simulink model "bicycle_kin_sim"  (R2020b)
settings: Solver=FixedStepAuto  StartTime=0.0  StopTime=inf  FixedStep=0.01  RelTol=1e-3
libraries: robotlib x8
settings Model: Creator=bascetta  LastModifiedBy=root
settings OptimizationCC: EnhancedBackFolding=on  PassReuseOutputArgsAs=Individual arguments  ZeroExternalMemoryAtStartup=off  ZeroInternalMemoryAtStartup=off  MaxStackSize=64  OptimizeBlockOrder=speed  DifferentSizesBufferReuse=on  OptimizationCustomize=off  EfficientTunableParamExpr=on
settings DebuggingCC: ParameterTunabilityLossMsg=error
settings HardwareCC: ProdBitPerPointer=32  ProdBitPerSizeT=32  ProdBitPerPtrDiffT=32  ProdLargestAtomicFloat=None  ProdIntDivRoundTo=Undefined  ProdEndianess=Unspecified  ProdWordSize=32  ProdHWDeviceType=Generic->Unspecified (assume 32-bit Generic)
settings SFSimCC: MATLABDynamicMemAlloc=off  SimTargetLang=C++
settings RTWCC: Description=Embedded Coder  SystemTargetFile=ert.tlc  HardwareBoard=Robot Operating System (ROS)  TLCOptions="-aInlineSetEventsForThisBaseRateFcn=TLC_FALSE -aSuppressMultiTaskScheduler=TLC_FALSE  -aRateBasedStepFcn=0"  GenCodeOnly=on  TemplateMakefile=ert_default_tmf  Toolchain=Catkin  TargetLang=C++
settings CodeAppCC: ForceParamTrailComments=on  IgnoreCustomStorageClasses=off  OperatorAnnotations=on  SimulinkDataObjDesc=on  SFDataObjDesc=on  InsertBlockDesc=on
settings ERTTargetCC: SupportContinuousTime=on  SupportVariableSizeSignals=on

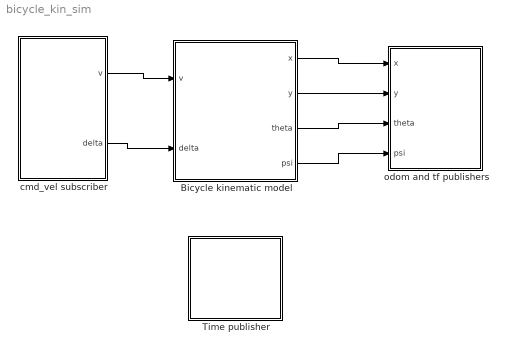
== system bicycle_kin_sim ==
  Bicycle kinematic model : Subsystem  mask{state0=[88, 182, 3.93], RCD=1.6, CFD=1.1}
      mask prompts: state0 "Initial conditions (x0, y0, theta0)"; RCD "Rear-Centre Distance"; CFD "Centre-Front Distance"
      mask TypeOptions RCD: Rear-Centre Distance/Value
      mask TypeOptions CFD: Centre-Front Distance/Value
  Time publisher : Subsystem
  cmd_vel subscriber : Subsystem
  odom and tf publishers : Subsystem  mask{simPublishRate=100}
      mask prompts: simPublishRate "Publising rate [Hz]"
  wires:
  Bicycle kinematic model/1(x) -> odom and tf publishers/1(x)
  Bicycle kinematic model/2(y) -> odom and tf publishers/2(y)
  Bicycle kinematic model/3(theta) -> odom and tf publishers/3(theta)
  cmd_vel subscriber/1(v) -> Bicycle kinematic model/1(v)
  cmd_vel subscriber/2(delta) -> Bicycle kinematic model/2(delta)
  Bicycle kinematic model/4(psi) -> odom and tf publishers/4(psi)

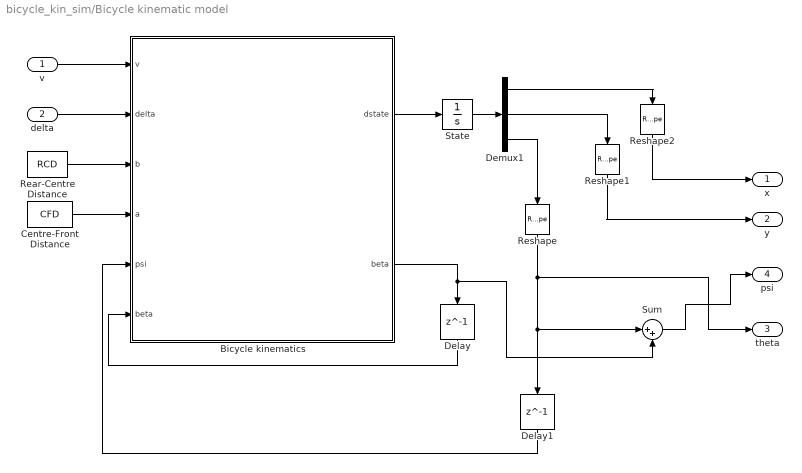
== system bicycle_kin_sim/Bicycle kinematic model ==
  v : Inport
  delta : Inport  Port=2
  Bicycle kinematics : MATLAB Function  TreatAsAtomicUnit=on
  Centre-Front Distance : Constant  Value=CFD
  Delay : Delay  DelayLength=1  InitialCondition=0
  Delay1 : Delay  DelayLength=1  InitialCondition=0
  Demux1 : Demux  Outputs=3
  Rear-Centre Distance : Constant  Value=RCD
  Reshape : Reshape
  Reshape1 : Reshape
  Reshape2 : Reshape
  State : Integrator  InitialCondition=state0
  Sum : Sum  Inputs=|++
  x : Outport  VectorParamsAs1DForOutWhenUnconnected=off
  y : Outport  Port=2  VectorParamsAs1DForOutWhenUnconnected=off
  theta : Outport  Port=3  VectorParamsAs1DForOutWhenUnconnected=off
  psi : Outport  Port=4  VectorParamsAs1DForOutWhenUnconnected=off
  wires:
  Bicycle kinematics/1(dstate) -> State/1
  State/1 -> Demux1/1
  Demux1/2 -> Reshape1/1
  Demux1/1 -> Reshape2/1
  delta/1 -> Bicycle kinematics/2(delta)
  v/1 -> Bicycle kinematics/1(v)
  Demux1/3 -> Reshape/1
  Bicycle kinematics/2(beta) -> Sum/2, Delay/1
  Rear-Centre Distance/1 -> Bicycle kinematics/3(b)
  Centre-Front Distance/1 -> Bicycle kinematics/4(a)
  Delay/1 -> Bicycle kinematics/6("beta ")
  Delay1/1 -> Bicycle kinematics/5(psi)
  Reshape/1 -> theta/1, Sum/1, Delay1/1
  Reshape1/1 -> y/1
  Reshape2/1 -> x/1
  Sum/1 -> psi/1

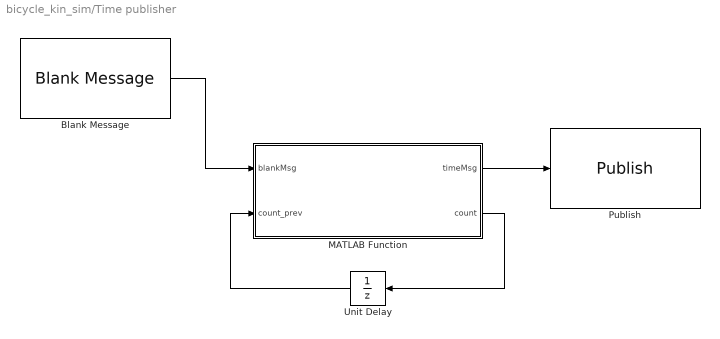
== system bicycle_kin_sim/Time publisher ==
  Blank Message : robotlib/Blank Message  messageClass=Message  entityType=rosgraph_msgs/Clock  messageType=rosgraph_msgs/Clock  SampleTime=0.01  legacyBusStruct=off
  MATLAB Function : MATLAB Function  TreatAsAtomicUnit=on
  Publish : robotlib/Publish  topicSource=Specify your own  topic=/clock  messageType=rosgraph_msgs/Clock  legacyBusStruct=off  messageQueueLength=1
  Unit Delay : UnitDelay  SampleTime=0.01  HasFrameUpgradeWarning=on
  wires:
  MATLAB Function/1(timeMsg) -> Publish/1
  Blank Message/1 -> MATLAB Function/1(blankMsg)
  MATLAB Function/2(count) -> Unit Delay/1
  Unit Delay/1 -> MATLAB Function/2(count_prev)

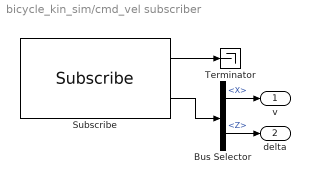
== system bicycle_kin_sim/cmd_vel subscriber ==
  Bus Selector : BusSelector  OutputSignals=Linear.X,Angular.Z
  Subscribe : robotlib/Subscribe  topicSource=Specify your own  topic=/cmd_vel  messageType=geometry_msgs/Twist  SampleTime=-1  legacyBusStruct=off  messageQueueLength=1
  Terminator : Terminator
  v : Outport
  delta : Outport  Port=2
  wires:
  Bus Selector/1 -> v/1  "<X>"
  Subscribe/2 -> Bus Selector/1
  Subscribe/1 -> Terminator/1
  Bus Selector/2 -> delta/1  "<Z>"

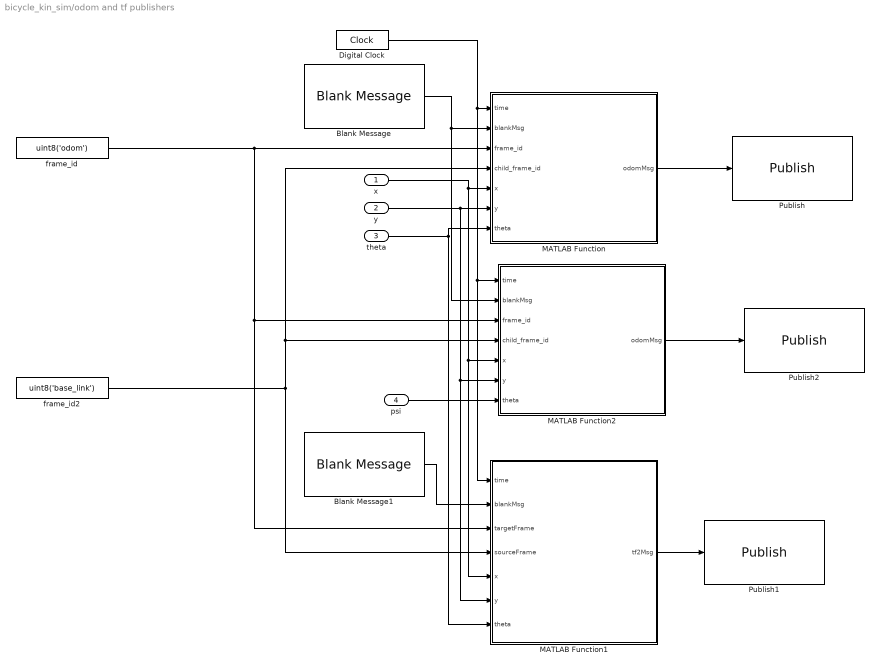
== system bicycle_kin_sim/odom and tf publishers ==
  x : Inport  SampleTime=1/simPublishRate
  y : Inport  Port=2  SampleTime=1/simPublishRate
  theta : Inport  Port=3  SampleTime=1/simPublishRate
  psi : Inport  Port=4  SampleTime=1/simPublishRate
  Blank Message : robotlib/Blank Message  messageClass=Message  entityType=nav_msgs/Odometry  messageType=nav_msgs/Odometry  SampleTime=1/simPublishRate  legacyBusStruct=off
  Blank Message1 : robotlib/Blank Message  messageClass=Message  entityType=tf2_msgs/TFMessage  messageType=tf2_msgs/TFMessage  SampleTime=1/simPublishRate  legacyBusStruct=off
  Digital Clock : DigitalClock  SampleTime=1/simPublishRate
  MATLAB Function : MATLAB Function  TreatAsAtomicUnit=on
  MATLAB Function1 : MATLAB Function  TreatAsAtomicUnit=on
  MATLAB Function2 : MATLAB Function  TreatAsAtomicUnit=on
  Publish : robotlib/Publish  topicSource=Specify your own  topic=/odom  messageType=nav_msgs/Odometry  legacyBusStruct=off  messageQueueLength=1
  Publish1 : robotlib/Publish  topicSource=Specify your own  topic=/tf  messageType=tf2_msgs/TFMessage  legacyBusStruct=off  messageQueueLength=1
  Publish2 : robotlib/Publish  topicSource=Specify your own  topic=/odom_chassis  messageType=nav_msgs/Odometry  legacyBusStruct=off  messageQueueLength=1
  frame_id : Constant  Value=uint8('odom')
  frame_id2 : Constant  Value=uint8('base_link')
  wires:
  theta/1 -> MATLAB Function/7(theta), MATLAB Function1/7(theta)
  y/1 -> MATLAB Function/6(y), MATLAB Function2/6(y), MATLAB Function1/6(y)
  x/1 -> MATLAB Function2/5(x), MATLAB Function1/5(x), MATLAB Function/5(x)
  Blank Message/1 -> MATLAB Function2/2(blankMsg), MATLAB Function/2(blankMsg)
  Digital Clock/1 -> MATLAB Function1/1(time), MATLAB Function2/1(time), MATLAB Function/1(time)
  MATLAB Function1/1(tf2Msg) -> Publish1/1
  Blank Message1/1 -> MATLAB Function1/2(blankMsg)
  frame_id2/1 -> MATLAB Function2/4(child_frame_id), MATLAB Function/4(child_frame_id), MATLAB Function1/4(sourceFrame)
  frame_id/1 -> MATLAB Function1/3(targetFrame), MATLAB Function2/3(frame_id), MATLAB Function/3(frame_id)
  MATLAB Function/1(odomMsg) -> Publish/1
  MATLAB Function2/1(odomMsg) -> Publish2/1
  psi/1 -> MATLAB Function2/7(theta)

== matlab function bicycle_kin_sim/Time publisher/MATLAB Function ==
  data: blankMsg input; count_prev input; timeMsg output Bus: SL_Bus_bicycle_kin_sim_rosgraph_msgs_Clock; count output
function [timeMsg,count] = generate_time_msg(blankMsg,count_prev)

time = count_prev*1e5;

blankMsg.Clock_.Sec = round(time*1e-9);
blankMsg.Clock_.Nsec = round(time-round(time));

count = count_prev+1;

timeMsg = blankMsg;

== matlab function bicycle_kin_sim/odom and tf publishers/MATLAB Function1 ==
  data: time input; blankMsg input; targetFrame input; sourceFrame input; x input; y input; tf2Msg output Bus: SL_Bus_bicycle_kin_sim_tf2_msgs_TFMessage; theta input
function tf2Msg = generate_tf2_msg(time,blankMsg, targetFrame, sourceFrame, x, y, theta)

% Set the number of transforms
blankMsg.Transforms_SL_Info.CurrentLength = uint32(1);


% Writing transform header
% Source frame is "base_link", target frame is "odom" 
blankMsg.Transforms(1).Header.Stamp.Sec = fix(time);
blankMsg.Transforms(1).Header.Stamp.Nsec = fix((time-fix(time))*1e9);
blankMsg.Transforms(1).Header.FrameId(1:length(targetFrame)) = targetFrame;
blankMsg.Transforms(1).Header.FrameId_SL_Info.CurrentLength = uint32(length(targetFrame));
blankMsg.Transforms(1).ChildFrameId(1:length(sourceFrame)) = sourceFrame;
blankMsg.Transforms(1).ChildFrameId_SL_Info.CurrentLength = uint32(length(sourceFrame));

% Writing transform traslation and rotation data
blankMsg.Transforms(1).Transform.Translation.X = x;
blankMsg.Transforms(1).Transform.Translation.Y = y;
blankMsg.Transforms(1).Transform.Translation.Z = 0;

rotation = eul2quat([0, 0, theta], 'ZYX');
blankMsg.Transforms(1).Transform.Rotation.X = rotation(1);
blankMsg.Transforms(1).Transform.Rotation.Y = rotation(2);
blankMsg.Transforms(1).Transform.Rotation.Z = rotation(3);
blankMsg.Transforms(1).Transform.Rotation.W = rotation(4);

tf2Msg = blankMsg;

== matlab function bicycle_kin_sim/Bicycle kinematic model/Bicycle kinematics ==
  data: v input; delta input; b input; a input; psi input; dstate output; beta output; beta input
function [dstate, beta] = bicycle_kinematics(v, delta, b, a, psi, beta)

l      = a + b ;

dx     = v*cos(beta + psi);
dy     = v*sin(beta + psi);
dpsi   = (v*cos(beta)*tan(delta))/l;

% There should be a limit to beta to be aligned to the assumptions
% (small slip angle)

beta = atan((b*tan(delta))/l);
%if (beta > 0.18 )
   % beta = 0.18;
%elseif(beta < -0.18)
    %beta = -0.18;
%end

dstate = [dx, dy, dpsi];

== matlab function bicycle_kin_sim/odom and tf publishers/MATLAB Function ==
  data: time input; blankMsg input; frame_id input; child_frame_id input; x input; y input; theta input; odomMsg output Bus: SL_Bus_bicycle_kin_sim_nav_msgs_Odometry
function odomMsg = generate_odom_msg(time,blankMsg,frame_id, child_frame_id,x,y,theta)

% Writing the message header
blankMsg.Header.Stamp.Sec = fix(time);
blankMsg.Header.Stamp.Nsec = fix((time-fix(time))*1e9);
blankMsg.Header.FrameId(1:length(frame_id)) = frame_id;
blankMsg.Header.FrameId_SL_Info.CurrentLength = uint32(length(frame_id));

% Write child frame id "base_link"
blankMsg.ChildFrameId(1:length(child_frame_id)) = child_frame_id;
blankMsg.ChildFrameId_SL_Info.CurrentLength = uint32(length(child_frame_id));
%blankMsg.ChildFrameId = child_frame_id;

% Write pose data
blankMsg.Pose.Pose.Position.X = x;
blankMsg.Pose.Pose.Position.Y = y;
blankMsg.Pose.Pose.Position.Z = 0;

orientation = eul2quat([0, 0, theta], 'ZYX');
blankMsg.Pose.Pose.Orientation.X = orientation(1);
blankMsg.Pose.Pose.Orientation.Y = orientation(2);
blankMsg.Pose.Pose.Orientation.Z = orientation(3);
blankMsg.Pose.Pose.Orientation.W = orientation(4);

odomMsg = blankMsg;

== matlab function bicycle_kin_sim/odom and tf publishers/MATLAB Function2 ==
  data: time input; blankMsg input; frame_id input; child_frame_id input; x input; y input; theta input; odomMsg output Bus: SL_Bus_bicycle_kin_sim_nav_msgs_Odometry
function odomMsg = generate_odom_msg(time,blankMsg,frame_id, child_frame_id,x,y,theta)

% Writing the message header
blankMsg.Header.Stamp.Sec = fix(time);
blankMsg.Header.Stamp.Nsec = fix((time-fix(time))*1e9);
blankMsg.Header.FrameId(1:length(frame_id)) = frame_id;
blankMsg.Header.FrameId_SL_Info.CurrentLength = uint32(length(frame_id));

% Write child frame id "base_link"
blankMsg.ChildFrameId(1:length(child_frame_id)) = child_frame_id;
blankMsg.ChildFrameId_SL_Info.CurrentLength = uint32(length(child_frame_id));
%blankMsg.ChildFrameId = child_frame_id;

% Write pose data
blankMsg.Pose.Pose.Position.X = x;
blankMsg.Pose.Pose.Position.Y = y;
blankMsg.Pose.Pose.Position.Z = 0;

orientation = eul2quat([0, 0, theta], 'ZYX');
blankMsg.Pose.Pose.Orientation.X = orientation(1);
blankMsg.Pose.Pose.Orientation.Y = orientation(2);
blankMsg.Pose.Pose.Orientation.Z = orientation(3);
blankMsg.Pose.Pose.Orientation.W = orientation(4);

odomMsg = blankMsg;
